simulink model "control_ppura"  (Simulink 7.7)
settings: Solver=ode4  StartTime=0.0  StopTime=400  FixedStep=0.05  RelTol=1e-3
values from neighbouring files (symbols this model uses):
  x_camino = u(1:long)    [calcula_indice.m]
  y_camino = u(long+1:2*long)    [calcula_indice.m]
undefined symbols (not defined in the file or in its folder): Dis_fija, kmp, r
libraries: simulink x2
settings Model: Creator=jaijicu1  LastModifiedBy=AValera
settings DebuggingCC: FcnCallInpInsideContextMsg=Enable All
settings SFSimCC: SimParseCustomCode=off
settings GRTTargetCC: CombineOutputUpdateFcns=on

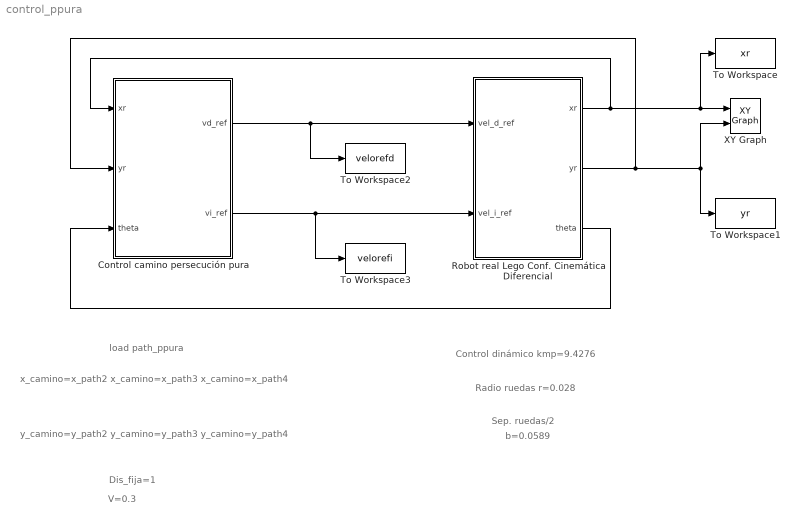
== system control_ppura ==
  note: Control dinámico
      | kmp=9.4276
  note: Sep. ruedas/2
  note: b=0.0589
  note: Radio ruedas
      | r=0.028
  note: x_camino=x_path2
      | x_camino=x_path3
      | x_camino=x_path4
  note: y_camino=y_path2
      | y_camino=y_path3
      | y_camino=y_path4
  note: Dis_fija=1
  note: V=0.3
  note: load path_ppura
  Control camino persecución pura : Subsystem
  Robot real Lego Conf. Cinemática Diferencial : Subsystem
  To Workspace : ToWorkspace  VariableName=xr  SampleTime=-1  SaveFormat=Array
  To Workspace1 : ToWorkspace  VariableName=yr  SampleTime=-1  SaveFormat=Array
  To Workspace2 : ToWorkspace  VariableName=velorefd  SampleTime=-1  SaveFormat=Array
  To Workspace3 : ToWorkspace  VariableName=velorefi  SampleTime=-1  SaveFormat=Array
  XY Graph : simulink/Sinks/XY Graph  SystemSampleTime=-1  xmin=-10  xmax=10  ymin=-10  ymax=10  st=-1
  wires:
  Control camino persecución pura/1(vd_ref) -> Robot real Lego Conf. Cinemática Diferencial/1(vel_d_ref), To Workspace2/1
  Control camino persecución pura/2(vi_ref) -> Robot real Lego Conf. Cinemática Diferencial/2(vel_i_ref), To Workspace3/1
  Robot real Lego Conf. Cinemática Diferencial/1(xr) -> XY Graph/1, To Workspace/1, Control camino persecución pura/1(xr)
  Robot real Lego Conf. Cinemática Diferencial/2(yr) -> XY Graph/2, To Workspace1/1, Control camino persecución pura/2(yr)
  Robot real Lego Conf. Cinemática Diferencial/3(theta) -> Control camino persecución pura/3(theta)

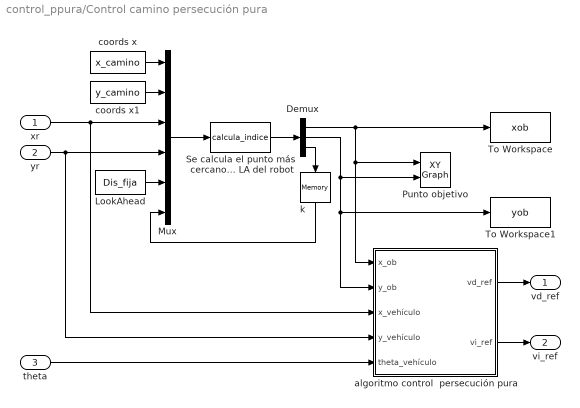
== system control_ppura/Control camino persecución pura ==
  xr : Inport
  yr : Inport  Port=2
  theta : Inport  Port=3
  Demux : Demux  Outputs=3
  LookAhead : Constant  Value=Dis_fija
  Mux : Mux  Inputs=6
  Punto objetivo : simulink/Sinks/XY Graph  SystemSampleTime=-1  xmin=-10  xmax=10  ymin=-10  ymax=10  st=-1
  Se calcula el punto más  cercano que está a una  distancia LA del robot : MATLABFcn  MATLABFcn=calcula_indice  OutputDimensions=3
  To Workspace : ToWorkspace  VariableName=xob  SampleTime=-1  SaveFormat=Array
  To Workspace1 : ToWorkspace  VariableName=yob  SampleTime=-1  SaveFormat=Array
  algoritmo control  persecución pura : Subsystem
  coords x : Constant  Value=x_camino
  coords x1 : Constant  Value=y_camino
  k : Memory  X0=1
  vd_ref : Outport
  vi_ref : Outport  Port=2
  wires:
  algoritmo control  persecución pura/2(vi_ref) -> vi_ref/1
  algoritmo control  persecución pura/1(vd_ref) -> vd_ref/1
  theta/1 -> algoritmo control  persecución pura/5(theta_vehículo)
  LookAhead/1 -> Mux/5
  Demux/3 -> k/1
  k/1 -> Mux/6
  Mux/1 -> Se calcula el punto más  cercano que está a una  distancia LA del robot/1
  coords x1/1 -> Mux/2
  coords x/1 -> Mux/1
  Se calcula el punto más  cercano que está a una  distancia LA del robot/1 -> Demux/1
  xr/1 -> algoritmo control  persecución pura/3(x_vehículo), Mux/3
  yr/1 -> algoritmo control  persecución pura/4(y_vehículo), Mux/4
  Demux/2 -> Punto objetivo/2, algoritmo control  persecución pura/2(y_ob), To Workspace1/1
  Demux/1 -> Punto objetivo/1, algoritmo control  persecución pura/1(x_ob), To Workspace/1

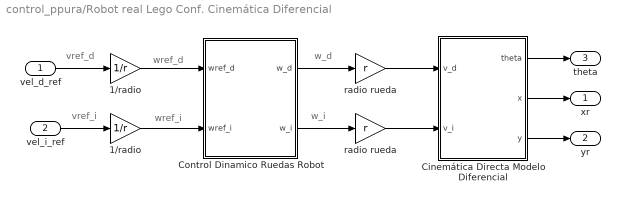
== system control_ppura/Robot real Lego Conf. Cinemática Diferencial ==
  note: w_d
  note: w_i
  note: vref_d
  note: wref_d
  note: vref_i
  note: wref_i
  vel_d_ref : Inport
  vel_i_ref : Inport  Port=2
  1/radio : Gain  Gain=1/r
  "1/radio " : Gain  Gain=1/r
  Cinemática Directa Modelo Diferencial : Subsystem
  Control Dinamico Ruedas Robot : Subsystem
  radio rueda : Gain  Gain=r
  "radio rueda " : Gain  Gain=r
  xr : Outport
  yr : Outport  Port=2
  theta : Outport  Port=3
  wires:
  Cinemática Directa Modelo Diferencial/3(y) -> yr/1
  Cinemática Directa Modelo Diferencial/2(x) -> xr/1
  vel_d_ref/1 -> 1/radio/1
  vel_i_ref/1 -> "1/radio "/1
  1/radio/1 -> Control Dinamico Ruedas Robot/1(wref_d)
  "1/radio "/1 -> Control Dinamico Ruedas Robot/2(wref_i)
  Control Dinamico Ruedas Robot/1(w_d) -> radio rueda/1
  Control Dinamico Ruedas Robot/2(w_i) -> "radio rueda "/1
  radio rueda/1 -> Cinemática Directa Modelo Diferencial/1(v_d)
  "radio rueda "/1 -> Cinemática Directa Modelo Diferencial/2(v_i)
  Cinemática Directa Modelo Diferencial/1(theta) -> theta/1

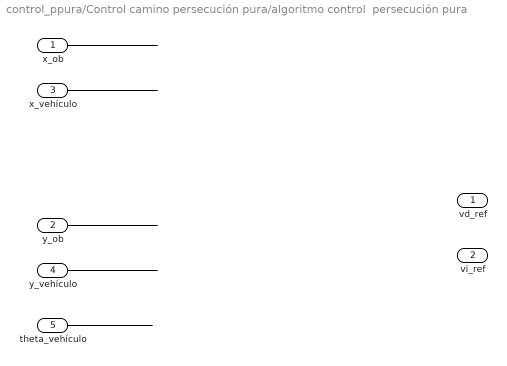
== system control_ppura/Control camino persecución pura/algoritmo control  persecución pura ==
  x_ob : Inport
  y_ob : Inport  Port=2
  x_vehículo : Inport  Port=3
  y_vehículo : Inport  Port=4
  theta_vehículo : Inport  Port=5
  vd_ref : Outport
  vi_ref : Outport  Port=2
  wires:
  y_vehículo/1 -> ?
  y_ob/1 -> ?
  x_vehículo/1 -> ?
  x_ob/1 -> ?
  theta_vehículo/1 -> ?

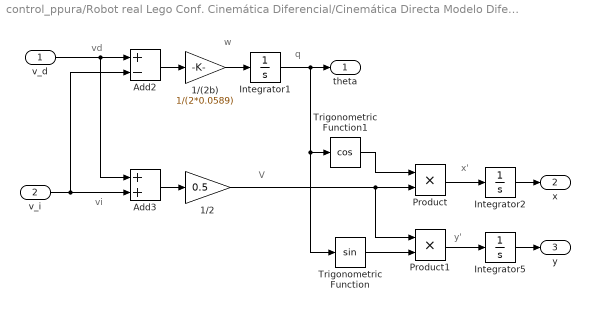
== system control_ppura/Robot real Lego Conf. Cinemática Diferencial/Cinemática Directa Modelo Diferencial ==
  note: w
  note: q
  note: y'
  note: x'
  note: V
  note: vi
  note: vd
  v_d : Inport
  v_i : Inport  Port=2
  1/(2b) : Gain  Gain=1/(2*0.0589)
  1/2 : Gain  Gain=0.5
  Add2 : Sum  Inputs=+-
  Add3 : Sum
  Integrator1 : Integrator  InitialCondition=pi/4
  Integrator2 : Integrator
  Integrator5 : Integrator
  Product : Product  RndMeth=Zero
  Product1 : Product  RndMeth=Zero
  Trigonometric Function : Trigonometry
  Trigonometric Function1 : Trigonometry  Operator=cos
  theta : Outport
  x : Outport  Port=2
  y : Outport  Port=3
  wires:
  Product1/1 -> Integrator5/1
  Product/1 -> Integrator2/1
  Integrator1/1 -> Trigonometric Function/1, Trigonometric Function1/1, theta/1
  1/(2b)/1 -> Integrator1/1
  Add2/1 -> 1/(2b)/1
  Add3/1 -> 1/2/1
  v_d/1 -> Add3/1, Add2/1
  v_i/1 -> Add2/2, Add3/2
  Trigonometric Function1/1 -> Product/1
  Trigonometric Function/1 -> Product1/2
  1/2/1 -> Product/2, Product1/1
  Integrator2/1 -> x/1
  Integrator5/1 -> y/1

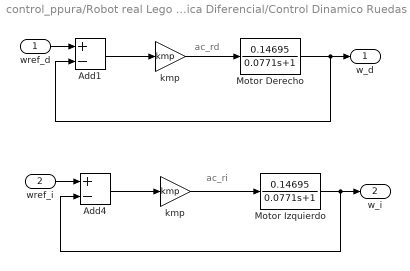
== system control_ppura/Robot real Lego Conf. Cinemática Diferencial/Control Dinamico Ruedas Robot ==
  note: ac_rd
  note: ac_ri
  wref_d : Inport
  wref_i : Inport  Port=2
  Add1 : Sum  Inputs=+-
  Add4 : Sum  Inputs=+-
  Motor Derecho : TransferFcn  Numerator=[0.14695]  Denominator=[0.0771 1]
  Motor Izquierdo : TransferFcn  Numerator=[0.14695]  Denominator=[0.0771 1]
  kmp : Gain  Gain=kmp
  "kmp " : Gain  Gain=kmp
  w_d : Outport
  w_i : Outport  Port=2
  wires:
  Motor Derecho/1 -> Add1/2, w_d/1
  Motor Izquierdo/1 -> Add4/2, w_i/1
  kmp/1 -> Motor Derecho/1
  Add1/1 -> kmp/1
  "kmp "/1 -> Motor Izquierdo/1
  Add4/1 -> "kmp "/1
  wref_d/1 -> Add1/1
  wref_i/1 -> Add4/1
